simulink model "tarefa13"  (R2022b)
settings: Solver=VariableStepAuto  StartTime=0.0  StopTime=30.0  RelTol=1e-3
values from neighbouring files (symbols this model uses):
  Cd = [0 1.092]    [lab11.m]    (also in lab13.m)
  d = -0.15    [lab11.m]    (also in lab13.m)
  F = [0.001 -0.382; 0.35 0.739]    [lab11.m]    (also in lab13.m)
  H = [0.35; 0.239]    [lab11.m]    (also in lab13.m)
  K = place(F,H,polos_dominantes)    [lab11.m]    (also in lab13.m)
  R = 1.25    [lab11.m]    (also in lab13.m)
  T0 = 0.377    [lab11.m]    (also in lab13.m)
  td = 15    [lab11.m]    (also in lab13.m)
settings Model: Creator=hugo_  LastModifiedBy=hugo_

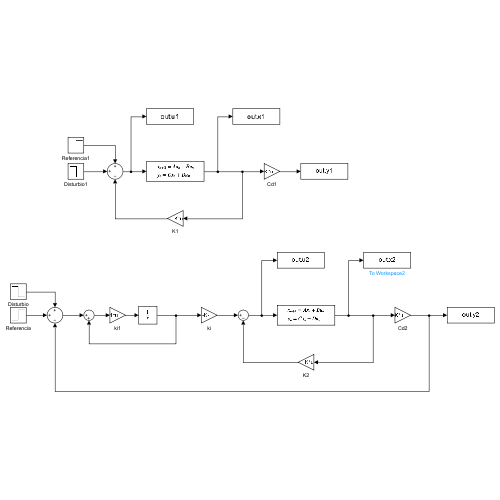
[thumbnail: Simulink's stored preview of the top-level diagram]
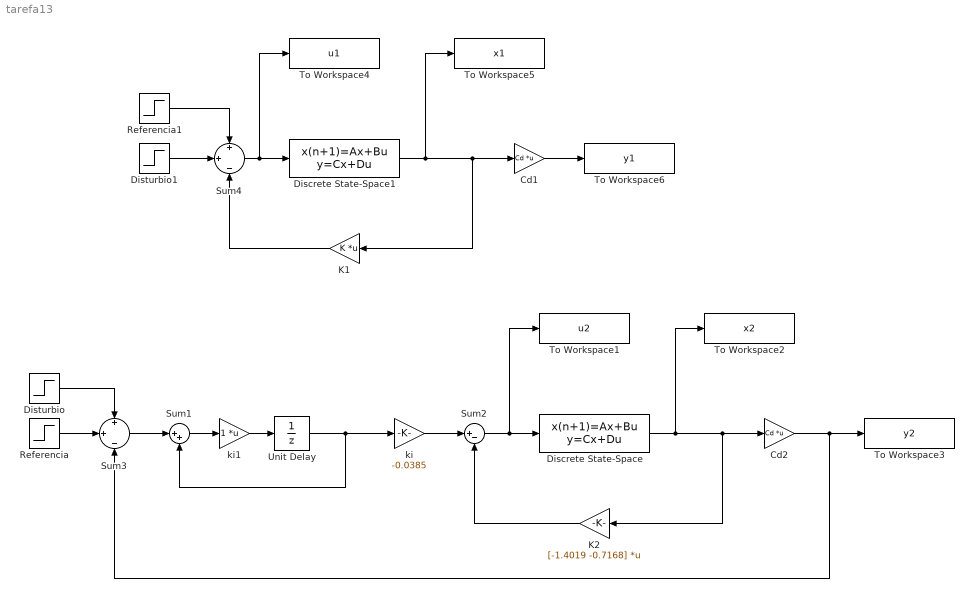
== system tarefa13 ==
  Cd1 : Gain  Gain=Cd  Multiplication=Matrix(K*u)
  Cd2 : Gain  Gain=Cd  Multiplication=Matrix(K*u)
  Discrete State-Space : DiscreteStateSpace  A=F  B=H  C=[1 0; 0 1]  D=[0;0]  SampleTime=T0
  Discrete State-Space1 : DiscreteStateSpace  A=F  B=H  C=[1 0; 0 1]  D=[0;0]  SampleTime=T0
  Disturbio : Step  Time=td  After=d  SampleTime=0
  Disturbio1 : Step  Time=td  After=d  SampleTime=0
  K1 : Gain  Gain=K  Multiplication=Matrix(K*u)
  K2 : Gain  Gain=[-1.4019 -0.7168]  Multiplication=Matrix(K*u)
  Referencia : Step  Time=0  After=R  SampleTime=0
  Referencia1 : Step  Time=0  After=R  SampleTime=0
  Sum1 : Sum  Inputs=|++
  Sum2 : Sum  Inputs=|+-
  Sum3 : Sum  Inputs=+|+|-
  Sum4 : Sum  Inputs=+|+|-
  To Workspace1 : ToWorkspace  VariableName=u2  SaveFormat=Timeseries  SampleTime=-1
  To Workspace2 : ToWorkspace  VariableName=x2  SaveFormat=Timeseries  SampleTime=-1
  To Workspace3 : ToWorkspace  VariableName=y2  SaveFormat=Timeseries  SampleTime=-1
  To Workspace4 : ToWorkspace  VariableName=u1  SaveFormat=Timeseries  SampleTime=-1
  To Workspace5 : ToWorkspace  VariableName=x1  SaveFormat=Timeseries  SampleTime=-1
  To Workspace6 : ToWorkspace  VariableName=y1  SaveFormat=Timeseries  SampleTime=-1
  Unit Delay : UnitDelay  SampleTime=T0  HasFrameUpgradeWarning=on
  ki : Gain  Gain=-0.0385
  ki1 : Gain  Multiplication=Matrix(K*u)
  wires:
  Discrete State-Space/1 -> To Workspace2/1, K2/1, Cd2/1
  Cd2/1 -> Sum3/3, To Workspace3/1
  Sum2/1 -> To Workspace1/1, Discrete State-Space/1
  K2/1 -> Sum2/2
  Unit Delay/1 -> ki/1, Sum1/2
  ki/1 -> Sum2/1
  Sum3/1 -> Sum1/1
  Referencia/1 -> Sum3/2
  Disturbio/1 -> Sum3/1
  Discrete State-Space1/1 -> To Workspace5/1, K1/1, Cd1/1
  Sum4/1 -> To Workspace4/1, Discrete State-Space1/1
  K1/1 -> Sum4/3
  Disturbio1/1 -> Sum4/2
  Referencia1/1 -> Sum4/1
  Cd1/1 -> To Workspace6/1
  ki1/1 -> Unit Delay/1
  Sum1/1 -> ki1/1
